simulink model "HIL"  (R2025b)
settings: Solver=FixedStepAuto  StartTime=0.0  StopTime=Inf  RelTol=1e-3  EnableMultiTasking=on
libraries: c280xlib x4
settings Model: ExtModeTrigDuration=8  Creator=USUARIO  LastModifiedBy=USUARIO
settings OptimizationCC: DefaultParameterBehavior=Inlined  DefaultUnderspecifiedDataType=single  EnhancedBackFolding=on  PassReuseOutputArgsAs=Individual arguments  MaxStackSize=1024  OptimizeBlockOrder=speed  DifferentSizesBufferReuse=on  OptimizationCustomize=off  EfficientTunableParamExpr=on
settings DebuggingCC: ParameterTunabilityLossMsg=error
settings HardwareCC: ProdBitPerChar=16.0  ProdBitPerInt=16.0  ProdBitPerPointer=32.0  ProdBitPerSizeT=32.0  ProdBitPerPtrDiffT=32.0  ProdLargestAtomicInteger=Integer  ProdLargestAtomicFloat=None  ProdWordSize=16.0  ProdLongLongMode=on  ProdHWDeviceType=Texas Instruments->C2000  HardwareBoardFeatureSet=SoCBlockset
settings SFSimCC: MATLABDynamicMemAlloc=off
settings RTWCC: SystemTargetFile=ert.tlc  HardwareBoard=TI Delfino F28379D LaunchPad  TemplateMakefile=ert_default_tmf  Toolchain=Texas Instruments Code Composer Studio (C2000)  CodeProfilingSaveOptions=MetricsOnly  Description=Embedded Coder
settings CodeAppCC: ForceParamTrailComments=on  IgnoreCustomStorageClasses=off  OperatorAnnotations=on  SimulinkDataObjDesc=on  SFDataObjDesc=on  InsertBlockDesc=on
settings ERTTargetCC: ExtModeTransport=4.0  ExtModeStaticAlloc=on  ExtModeAutomaticAllocSize=off  ExtModeStaticAllocSize=10000.0  ExtModeMexFile=ext_xcp  ExtModeIntrfLevel=Level2 - Open  CodeReplacementLibrary=TI C28x

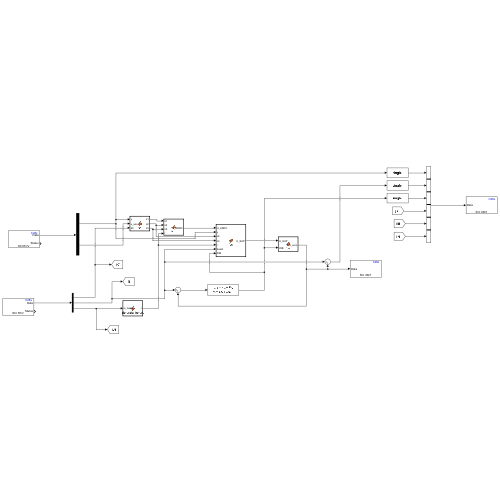
[thumbnail: Simulink's stored preview of the top-level diagram]
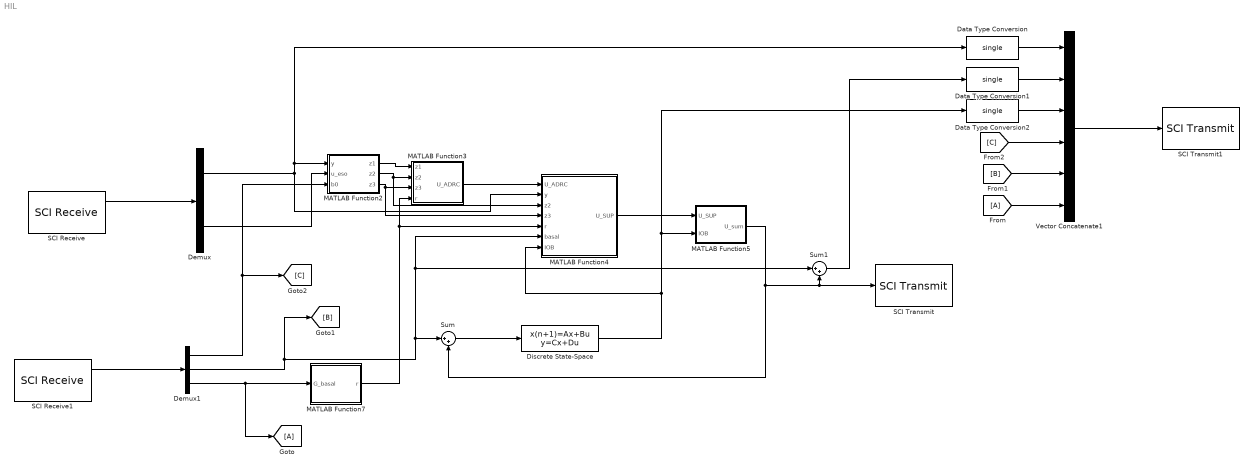
== system HIL ==
  Data Type Conversion : DataTypeConversion  OutDataTypeStr=single  SaturateOnIntegerOverflow=off  RndMeth=Floor
  Data Type Conversion1 : DataTypeConversion  OutDataTypeStr=single  SaturateOnIntegerOverflow=off  RndMeth=Floor
  Data Type Conversion2 : DataTypeConversion  OutDataTypeStr=single  SaturateOnIntegerOverflow=off  RndMeth=Floor
  Demux : Demux  Outputs=2
  Demux1 : Demux  Outputs=3
  Discrete State-Space : DiscreteStateSpace  A=|  B=|  C=[1 1]  D=0  InitialCondition=[0;0]
      A=|
      | [0.98383213 0;
      |      0.01603646 0.98383213]
      B=|
      | [0.01653157;
      |      0.00013437]
  From : From
  Goto : Goto
  MATLAB Function2 : MATLAB Function  TreatAsAtomicUnit=on
  MATLAB Function3 : MATLAB Function  TreatAsAtomicUnit=on
  MATLAB Function4 : MATLAB Function  TreatAsAtomicUnit=on
  MATLAB Function5 : MATLAB Function  TreatAsAtomicUnit=on
  MATLAB Function7 : MATLAB Function  TreatAsAtomicUnit=on
  SCI Receive : c280xlib/SCI Receive  Priority=2  sciModule=A  dataHead='S'  headerCheckMaxCount=16  dataTail='E'  dataType=single  dataLenOptions=Length via dialog  dataDim=4  maxDataLength=1  initValue=0  errOption=Output the last received value  errValue=0  sampleTime=1  blockingMode=on  timeOut=inf  outputStatus=on
      settings: LibrarySourceBlock=c2837xDlib/SCI Receive
  SCI Receive1 : c280xlib/SCI Receive  Priority=2  sciModule=B  dataHead='S'  headerCheckMaxCount=16  dataTail='E'  dataType=single  dataLenOptions=Length via dialog  dataDim=3  maxDataLength=1  initValue=0  errOption=Output the last received value  errValue=0  sampleTime=0.1  blockingMode=on  timeOut=inf  outputStatus=on
      settings: LibrarySourceBlock=c2837xDlib/SCI Receive
  SCI Transmit : c280xlib/SCI Transmit  sciModule=A  dataHead='R'  dataTail='E'  frameSize=1  blockingMode=on  outputStatus=off
      settings: LibrarySourceBlock=c2837xDlib/SCI Transmit
  SCI Transmit1 : c280xlib/SCI Transmit  sciModule=B  dataHead='S'  dataTail='E'  frameSize=1  blockingMode=on  outputStatus=off
      settings: LibrarySourceBlock=c2837xDlib/SCI Transmit
  Sum : Sum  Inputs=|++
  Sum1 : Sum  Inputs=|++
  Vector Concatenate1 : Concatenate  NumInputs=6
  wires:
  MATLAB Function4/1(U_SUP) -> MATLAB Function5/1(U_SUP)
  MATLAB Function3/1(U_ADRC) -> MATLAB Function4/1(U_ADRC)
  MATLAB Function2/1(z1) -> MATLAB Function3/1(z1)
  MATLAB Function2/2(z2) -> MATLAB Function4/3(z2), MATLAB Function3/2(z2)
  MATLAB Function2/3(z3) -> MATLAB Function4/4(z3), MATLAB Function3/3(z3)
  Demux/2 -> MATLAB Function2/2(u_eso)
  SCI Receive/1 -> Demux/1
  Discrete State-Space/1 -> Data Type Conversion2/1, MATLAB Function5/2(IOB), MATLAB Function4/7(IOB)
  Sum/1 -> Discrete State-Space/1
  Demux/1 -> Data Type Conversion/1, MATLAB Function2/1(y), MATLAB Function4/2(y)
  MATLAB Function5/1(U_sum) -> SCI Transmit/1, Sum1/2, Sum/2
  Vector Concatenate1/1 -> SCI Transmit1/1
  Data Type Conversion/1 -> Vector Concatenate1/1
  Sum1/1 -> Data Type Conversion1/1
  Data Type Conversion1/1 -> Vector Concatenate1/2
  Data Type Conversion2/1 -> Vector Concatenate1/3
  Demux1/1 -> [C], MATLAB Function2/3(b0)
  SCI Receive1/1 -> Demux1/1
  Demux1/2 -> [B], MATLAB Function4/6(basal), Sum1/1, Sum/1
  MATLAB Function7/1(r) -> MATLAB Function3/4(r), MATLAB Function4/5(r)
  Demux1/3 -> MATLAB Function7/1(G_basal), Goto/1
  From/1 -> Vector Concatenate1/6
  [B] -> Vector Concatenate1/5
  [C] -> Vector Concatenate1/4

== matlab function HIL/MATLAB Function2 ==
  data: y input; z1 output; u_eso input; z2 output; z3 output; b0 input
function [z1,z2,z3] = fcn(y,u_eso,b0)

persistent z

if isempty(z)
    z = single([0;0;0]);
end

y     = single(y);
u_eso = single(u_eso);

Ad = single([ ...
     0.6163,  0.7984,  0.4312;
    -0.0540,  0.9711,  0.9901;
    -0.0026, -0.0014,  0.9995]);

Bd = single([ ...
    -0.0327,  0.3837;
    -0.0792,  0.0540;
     0.0000,  0.0026]);

z = Ad*z + Bd*[u_eso; y];

z1 = z(1);
z2 = z(2);
z3 = z(3);

end

== matlab function HIL/MATLAB Function3 ==
  data: z1 input; U_ADRC output; z2 input; z3 input; r input
function U_ADRC = fcn(z1, z2, z3, r)

z1 = single(z1);
z2 = single(z2);
z3 = single(z3);
r  = single(r);

b0 = single(-0.08);
Kp = single(0.00096570645);
Kd = single(0.08222222);

e  = r - z1;
de = -z2;

u01 = Kp*e + Kd*de;

U_ADRC = (u01 - z3) / b0;

% Saturación [-1, 7]
limiteInferior = single(-1.2);

if U_ADRC > single(7)
    U_ADRC = single(7);
elseif U_ADRC < limiteInferior
    U_ADRC = limiteInferior;
end

end

== matlab function HIL/MATLAB Function4 ==
  data: U_ADRC input; U_SUP output; y input; z2 input; z3 input; r input; basal input; IOB input
function U_SUP = fcn(U_ADRC,y,z2,z3,r,basal,IOB)

U_ADRC = single(U_ADRC);
y      = single(y);
z2     = single(z2);
z3     = single(z3);
r      = single(r);
basal  = single(basal);
IOB    = single(IOB);

deadband = single(15);

G_low  = single(-45);
G_high = single(20);

z3_noise = single(0.08);
z3_meal  = single(0.10);

z2_down1 = single(-0.25);
z2_down2 = single(-0.60);

IOB_soft = single(3.5);
IOB_med  = single(4.5);
IOB_high = single(5.2);

U_SUP = U_ADRC;

% 1. Glucosa baja
if y < G_low

    U_SUP = single(-0.95)*basal;
    return

end

% 2. Limitacion por IOB
if U_SUP > single(0)

    if IOB >= IOB_high

        U_SUP = single(0.20)*U_SUP;

    elseif IOB >= IOB_med

        U_SUP = single(0.45)*U_SUP;

    elseif IOB >= IOB_soft

        U_SUP = single(0.70)*U_SUP;

    end

end

% 3. Perturbacion detectada
if z3 > z3_meal
    return
end

% 4. Cerca de referencia
if abs(y-r) < deadband && abs(z3) < z3_noise

    if abs(U_ADRC) < single(0.8)
        U_SUP = single(0);
    end

end

% 5. Glucosa descendiendo
if z2 < z2_down1 && U_SUP > single(0)

    U_SUP = single(0.75)*U_SUP;

end

% 6. Caida fuerte
if z2 < z2_down2 && y < single(-25)

    U_SUP = single(-0.95)*basal;
    return

end

% 7. Glucosa alta
if y > G_high
    return
end

end

== matlab function HIL/MATLAB Function5 ==
  data: U_SUP input; U_sum output; IOB input
function U_sum = fcn(U_SUP,IOB)

persistent relay_high

if isempty(relay_high)
    relay_high = false;
end

U_SUP = single(U_SUP);
IOB   = single(IOB);

% =========================================================
% 1. Señal negativa permitida
% =========================================================
if U_SUP > single(0)
    U_NEG = single(0);
elseif U_SUP < single(-1000)
    U_NEG = single(-1000);
else
    U_NEG = U_SUP;
end

% =========================================================
% 2. Relay con histéresis según IOB
% =========================================================
if relay_high == false

    if IOB >= single(5.5)
        relay_high = true;
    end

else

    if IOB <= single(4.4)
        relay_high = false;
    end

end

% =========================================================
% 3. Selección SAFE
% =========================================================
if relay_high
    U_sum = U_NEG;
else
    U_sum = U_SUP;
end

% =========================================================
% 4. Saturación final de la acción correctiva
% =========================================================
if U_sum > single(2.5)
    U_sum = single(2.5);
elseif U_sum < single(-1.4997)
    U_sum = single(-1.4997);
end

end

== matlab function HIL/MATLAB Function7 ==
  data: G_basal input; r output
function r = referencia_horaria( G_basal)



end
